simulink model "firstSym"  (R2017a)
settings: Solver=VariableStepAuto  StartTime=0.0  StopTime=2  MaxStep=0.01  RelTol=1e-4  EnableMultiTasking=on
PreLoadFcn:
  | datas
undefined symbols (not defined in the file or in its folder): Fx
settings Model: Creator=edoardoghini  LastModifiedBy=edoardoghini
settings DataIOCC: LimitDataPoints=on  SaveOutput=off  SaveTime=off
settings OptimizationCC: ExpressionDepthLimit=2147483647  LifeSpan=1
settings DebuggingCC: UnderspecifiedInitializationDetection=Classic  MergeDetectMultiDrivingBlocksExec=none  FcnCallInpInsideContextMsg=warning  AllowSymbolicDim=off  StateNameClashWarn=warning  SFUnexpectedBacktrackingDiag=warning  SFNoUnconditionalDefaultTransitionDiag=warning  SFExecutionAtInitializationDiag=none
settings GRTTargetCC: TargetLangStandard=C89/C90 (ANSI)  GeneratePreprocessorConditionals=Disable all  CombineOutputUpdateFcns=off  GRTInterface=on

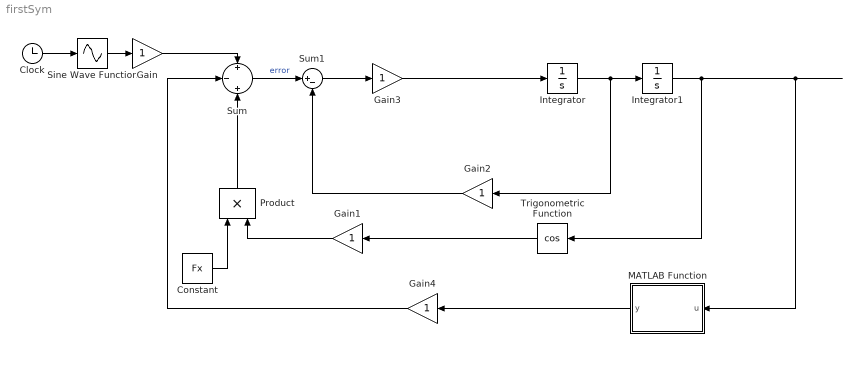
== system firstSym ==
  Clock : Clock
  Constant : Constant  Value=Fx
  Gain{,1..4} (5 alike) : Gain
  Integrator : Integrator
  Integrator1 : Integrator
  MATLAB Function : MATLAB Function  TreatAsAtomicUnit=on
  Product : Product
  Sine Wave Function : Sin  TimeSource=Use external signal  Frequency=3  SampleTime=0
  Sum : Sum  Inputs=+|-|+
  Sum1 : Sum  Inputs=|+-
  Trigonometric Function : Trigonometry  Operator=cos
  wires:
  Clock/1 -> Sine Wave Function/1
  Gain/1 -> Sum/1
  Sine Wave Function/1 -> Gain/1
  Sum/1 -> Sum1/1  "error"
  Sum1/1 -> Gain3/1
  Gain3/1 -> Integrator/1
  Integrator/1 -> Gain2/1, Integrator1/1
  Integrator1/1 -> Trigonometric Function/1, MATLAB Function/1(u)
  Gain2/1 -> Sum1/2
  Gain1/1 -> Product/2
  Product/1 -> Sum/3
  Constant/1 -> Product/1
  Trigonometric Function/1 -> Gain1/1
  MATLAB Function/1(y) -> Gain4/1
  Gain4/1 -> Sum/2

== matlab function firstSym/MATLAB Function ==
  data: u input; y output
function y = fcn(u)

y = u;
